simulink model "roll_control_loop"  (R2019b)
settings: Solver=VariableStepAuto  StartTime=0.0  StopTime=50  FixedStep=1e-4  RelTol=1e-6
values from neighbouring files (symbols this model uses):
  Kinner = 0.003    [main.m]
  Kouter = 2.72    [main.m]
  Ld = 0.1568*U^2    (= 8179.716608)    [main.m]
  Lp = -0.07946*U    (= -18.148664)    [main.m]
  tauSensor = 0.01    [main.m]
  tauServo = 0.1    [main.m]
libraries: simulink_extras x1, simulink x1
settings Model: Creator=guy-m  LastModifiedBy=guy-m

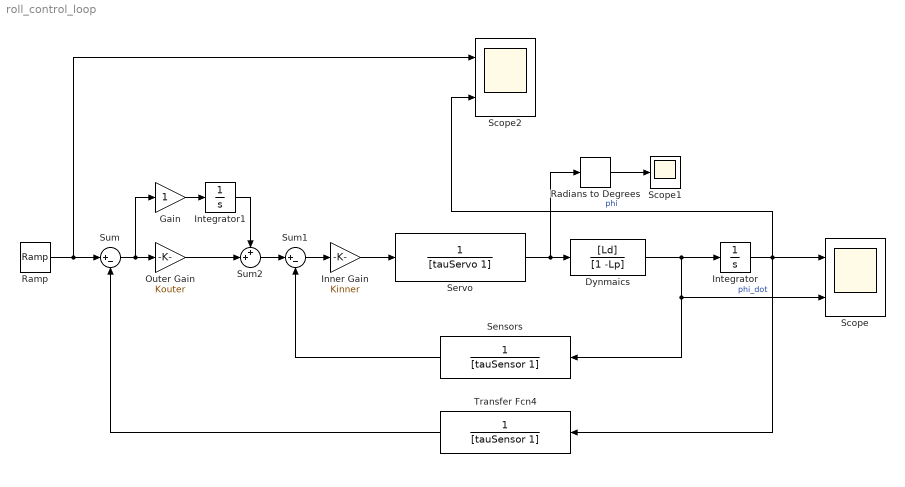
== system roll_control_loop ==
  Dynmaics : TransferFcn  Numerator=[Ld]  Denominator=[1 -Lp]
  Gain : Gain
  Inner Gain : Gain  Gain=Kinner
  Integrator : Integrator
  Integrator1 : Integrator
  Outer Gain : Gain  Gain=Kouter
  Radians to Degrees : simulink_extras/Transformations/Radians to Degrees
  Ramp : simulink/Sources/Ramp  slope=0.5  start=0  InitialOutput=0
  Scope : Scope  NumInputPorts=2
  Scope1 : Scope
  Scope2 : Scope  NumInputPorts=2
  Sensors : TransferFcn  Numerator=1  Denominator=[tauSensor 1]
  Servo : TransferFcn  Numerator=1  Denominator=[tauServo 1]
  Sum : Sum  Inputs=|+-
  Sum1 : Sum  Inputs=|+-
  Sum2 : Sum  Inputs=++|
  Transfer Fcn4 : TransferFcn  Numerator=1  Denominator=[tauSensor 1]
  wires:
  Ramp/1 -> Scope2/1, Sum/1
  Sum/1 -> Gain/1, Outer Gain/1
  Sum1/1 -> Inner Gain/1
  Dynmaics/1 -> Sensors/1, Scope/2, Integrator/1  "phi_dot"
  Integrator/1 -> Scope2/2, Scope/1, Transfer Fcn4/1  "phi"
  Sensors/1 -> Sum1/2
  Transfer Fcn4/1 -> Sum/2
  Inner Gain/1 -> Servo/1
  Outer Gain/1 -> Sum2/2
  Servo/1 -> Radians to Degrees/1, Dynmaics/1
  Radians to Degrees/1 -> Scope1/1
  Gain/1 -> Integrator1/1
  Sum2/1 -> Sum1/1
  Integrator1/1 -> Sum2/1
